simulink model "PID_controller_gaussian_noise"  (R2024b)
settings: Solver=VariableStepAuto  StartTime=0.0  StopTime=60  RelTol=1e-3
values from neighbouring files (symbols this model uses):
  Kd = 0.1    [calculate_metrics_controlers.m]
  Ki = 0.1    [calculate_metrics_controlers.m]
  Kp = 2.5    [calculate_metrics_controlers.m]
  SATURATION = 22    [calculate_metrics_controlers.m]
libraries: slpidlib x1
settings Model: Creator=gonzaloma  LastModifiedBy=gonzaloma

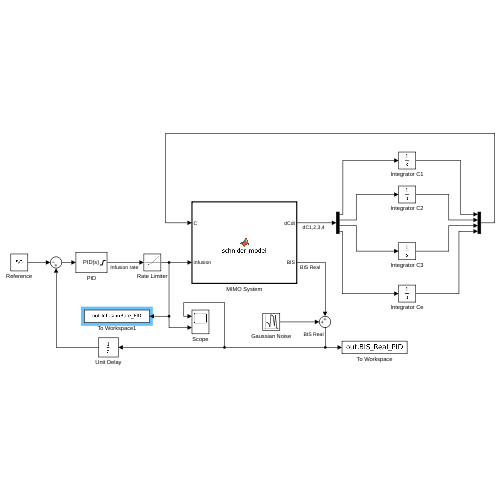
[thumbnail: Simulink's stored preview of the top-level diagram]
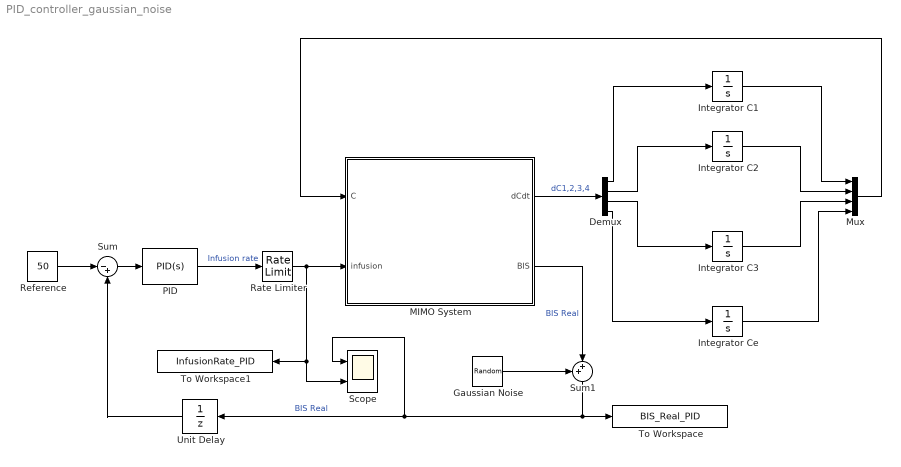
== system PID_controller_gaussian_noise ==
  Demux : Demux
  Gaussian Noise : RandomNumber  Seed=13  SampleTime=1/60
  Integrator C1 : Integrator  InitialCondition=1.7547
  Integrator C2 : Integrator  InitialCondition=0.17
  Integrator C3 : Integrator  InitialCondition=0.0759
  Integrator Ce : Integrator  InitialCondition=0.1658
  MIMO System : MATLAB Function  TreatAsAtomicUnit=on
  Mux : Mux
  PID : slpidlib/PID Controller  Controller=PID  Form=Parallel  TimeDomain=Continuous-time  UseExternalTs=off  SampleTime=1/60  IntegratorMethod=Forward Euler  FilterMethod=Forward Euler  ControllerParametersSource=internal  P=Kp  I=Ki  UseKiTs=off  D=Kd  UseExternalDerivativeSource=off  N=100  UseFilter=on  TunerSelectOption=Transfer Function Based (PID Tuner App)  InitialConditionSource=internal  InitialConditionForIntegrator=0  InitialConditionForFilter=0  DifferentiatorICPrevScaledInput=0  ExternalReset=none  TrackingMode=off  Kt=1  LimitOutput=on  SatLimitsSource=internal  UpperSaturationLimit=SATURATION  LowerSaturationLimit=0  LinearizeAsGain=on  AntiWindupMode=none  Kb=1  LimitIntegrator=off  UpperIntegratorSaturationLimit=inf  LowerIntegratorSaturationLimit=-inf  POutMin=[]  POutMax=[]  IOutMin=[]  IOutMax=[]  DOutMin=[]  DOutMax=[]  NOutMin=[]  NOutMax=[]  SumOutMin=[]  SumOutMax=[]  SaturationOutMin=[]  SaturationOutMax=[]  PParamMin=[]  PParamMax=[]  IParamMin=[]  IParamMax=[]  DParamMin=[]  DParamMax=[]  NParamMin=[]  NParamMax=[]  KbParamMin=[]  KbParamMax=[]  KtParamMin=[]  KtParamMax=[]  KbOutMin=[]  KbOutMax=[]  KtOutMin=[]  KtOutMax=[]  IntegratorOutMin=[]  IntegratorOutMax=[]  FilterOutMin=[]  FilterOutMax=[]  SumI1OutMin=[]  SumI1OutMax=[]  SumI2OutMin=[]  SumI2OutMax=[]  SumI3OutMin=[]  SumI3OutMax=[]  SumI4OutMin=[]  SumI4OutMax=[]  SumDOutMin=[]  SumDOutMax=[]  DifferentiatorOutMin=[]  DifferentiatorOutMax=[]  FilterDiffOutCoefMin=[]  FilterDiffOutCoefMax=[]  ReciprocalOutMin=[]  ReciprocalOutMax=[]  SumDenOutMin=[]  SumDenOutMax=[]  SumNumOutMin=[]  SumNumOutMax=[]  DivideOutMin=[]  DivideOutMax=[]  UdiffTsProdOutMin=[]  UdiffTsProdOutMax=[]  NTsProdOutMin=[]  NTsProdOutMax=[]  UintegralTsProdOutMin=[]  UintegralTsProdOutMax=[]  UngainTsProdOutMin=[]  UngainTsProdOutMax=[]  ClampingZeroOutDataTypeStr=Inherit: Inherit via back propagation  ClampingZeroOutMin=[]  ClampingZeroOutMax=[]  FilterDenConstantOutDataTypeStr=Inherit: Inherit via back propagation  FilterDenConstantOutMin=[]  FilterDenConstantOutMax=[]  PCopyOutDataTypeStr=Inherit: Inherit via back propagation  PCopyOutMin=[]  PCopyOutMax=[]  NCopyOutDataTypeStr=Inherit: Inherit via back propagation  NCopyOutMin=[]  NCopyOutMax=[]  IntegratorContinuousStateAttributes=''  IntegratorStateMustResolveToSignalObject=off  IntegratorRTWStateStorageClass=Auto  FilterContinuousStateAttributes=''  FilterStateMustResolveToSignalObject=off  FilterRTWStateStorageClass=Auto  ParallelPVariant=InternalParameters  IdealPVariant=Disabled  IVariant=InternalParameters  DVariant=InternalParameters  IntegratorVariant=Continuous  SatVariant=Enabled  AWVariant=Passthrough  PCopyVariant=Disabled  TRVariant=Disabled  FdbkBlocksVariant=Forward  IdealPFdbkVariant=Disabled  SatFdbkVariant=Disabled  DerivativeFilterVariant=ContFilter  NVariant=InternalParameters  NCopyVariant=Disabled  FilterICVariant=InternalICsFilter  IntegratorICVariant=InternalICs  ExternalResetVariant=Disabled  TRSumVariant=Passthrough  SumFdbkVariant=Disabled  SumVariant=Sum_PID  TsampFilterVariant=InternalTs  TsampNgainVariant=Passthrough  TsampIntegralVariant=Disabled_SignalSpec  ExternalSaturationOutDataTypeStr=Inherit: Same as second input  DerivativeSourceVariant=ErrorSignal  PreIntVariant=InternalPreInt
  Rate Limiter : RateLimiter  RisingSlewLimit=2  FallingSlewLimit=-2
  Reference : Constant  Value=50
  Scope : Scope  NumInputPorts=2
  Sum : Sum  Inputs=|-+
  Sum1 : Sum  Inputs=++|
  To Workspace : ToWorkspace  VariableName=BIS_Real_PID  SampleTime=-1
  To Workspace1 : ToWorkspace  VariableName=InfusionRate_PID  SampleTime=-1
  Unit Delay : UnitDelay  InitialCondition=100  SampleTime=1/60  HasFrameUpgradeWarning=on
  wires:
  Sum/1 -> PID/1
  MIMO System/1(dCdt) -> Demux/1  "dC1,2,3,4"
  Integrator C2/1 -> Mux/2
  Demux/3 -> Integrator C3/1
  Demux/4 -> Integrator Ce/1
  Integrator C3/1 -> Mux/3
  Integrator Ce/1 -> Mux/4
  Mux/1 -> MIMO System/1(C)
  Demux/1 -> Integrator C1/1
  Integrator C1/1 -> Mux/1
  Demux/2 -> Integrator C2/1
  PID/1 -> Rate Limiter/1  "Infusion rate"
  Unit Delay/1 -> Sum/2
  Rate Limiter/1 -> MIMO System/2(infusion), To Workspace1/1, Scope/2
  Reference/1 -> Sum/1
  Gaussian Noise/1 -> Sum1/1
  MIMO System/2(BIS) -> Sum1/2  "BIS Real"
  Sum1/1 -> To Workspace/1, Unit Delay/1, Scope/1  "BIS Real"

== matlab function PID_controller_gaussian_noise/MIMO System ==
  settings: updateMethod=CONTINUOUS
  data: dCdt output size=[4, 1]; C input; infusion input; BIS output
function [dCdt, BIS] = schnider_model(C, infusion)
%#codegen

% Inputs:
%   t        - tiempo actual
%   C        - estado actual [C1; C2; C3; Ce]
%   infusion - tasa de infusión actual (u)
%   params   - estructura con parámetros

% Outputs:
%   dCdt - derivadas del estado
%   BIS  - salida (nivel BIS)

% Parametros
age = 28; % Age in years
weight = 60; % Weight in kg
height = 164; % Height in cm
gender = "M"; % Gender (M = Male; F = Female)

% Lean body mass calculation based on gender
if strcmp(gender, "M")
    LBM = (1.1 * weight) - 128 * (weight / height)^2; % Lean body mass (kg)
else
    LBM = (1.07 * weight) - 148 * (weight / height)^2; % Lean body mass (kg)
end

Ce50 = 4.93; % Effect site concentration for BIS 50 (mg/L)
gamma = 2.46; % Slope of the concentration-response curve

% Pharmacokinetic parameters of the Schnider model
V1 = 4.27; % Central compartment volume (L)
V2 = 18.9 - 0.391 * (age - 53); % Rapid peripheral compartment volume (L)
V3 = 238; % Slow peripheral compartment volume (L)

CL1 = 1.89 + ((weight - 77) * 0.0456) + ((LBM - 59) * (-0.0681)) + ((height - 177) * 0.0264); % Clearance of the central compartment (L/min)
CL2 = 1.29 - 0.024 * (age - 53); % Clearance between central and rapid peripheral compartment (L/min)
CL3 = 0.836; % Clearance between central and slow peripheral compartment (L/min)

% Transfer rate constants (calculated from clearances and volumes)
k10 = CL1 / V1;
k12 = CL2 / V1;
k13 = CL3 / V1;
k21 = CL2 / V2;
k31 = CL3 / V3;

% Pharmacodynamic (PD) effect-site parameters
ke0 = 0.456; % Rate constant for equilibrium between plasma and effect site (1/min)

% Additional parameters
BIS_base = 100; % Baseline BIS value (no drug effect)

% Dinámica PK (modelo de Schnider)
dCdt = zeros(4,1);
dCdt(1) = (infusion / V1) ...
          - k10*C(1) ...
          - k12*C(1) + k21*C(2) ...
          - k13*C(1) + k31*C(3);
      
dCdt(2) = k12*C(1) - k21*C(2);
dCdt(3) = k13*C(1) - k31*C(3);
dCdt(4) = ke0 * (C(1) - C(4)); % Sitio de efecto (Ce)

% Salida BIS
BIS = BIS_base * (Ce50^gamma) / ...
      (Ce50^gamma + C(4)^gamma);
